simulink model "LLC2"  (R2018a)
settings: Solver=VariableStepAuto  StartTime=0.0  StopTime=0.01  RelTol=1e-3
undefined symbols (not defined in the file): Lm
libraries: powerlib x39, powerlib_meascontrol x2
settings Model: Creator=sy167  LastModifiedBy=sy167

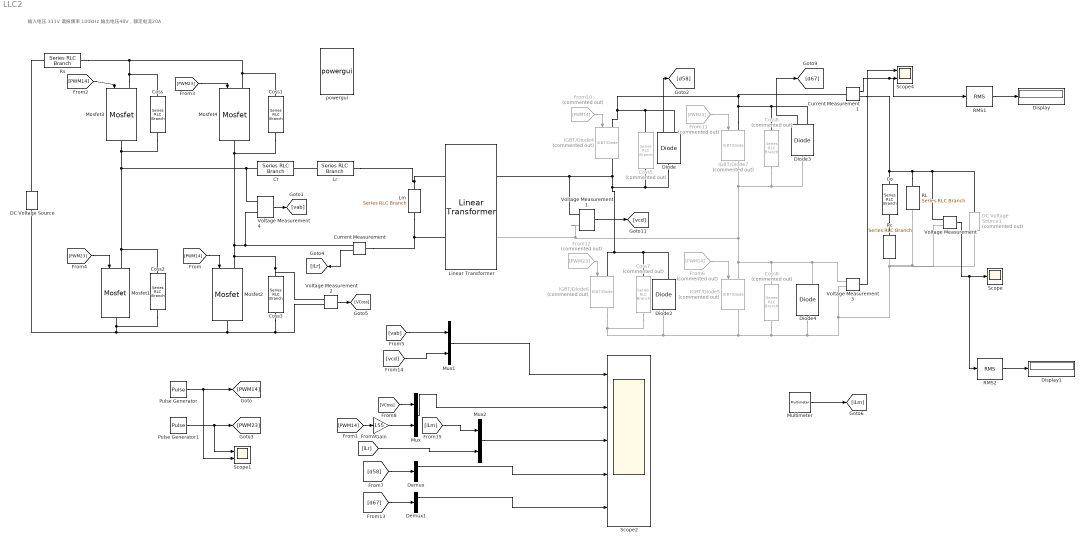
== system LLC2 ==
  note: 输入电压 311V 谐振频率 100kHz 输出电压48V，额定电流20A
  Co : powerlib/Elements/Series RLC Branch  LConnTagsString=__new0  RConnTagsString=__new0  BranchType=C  Resistance=1  Inductance=72e-6  SetiL0=off  InitialCurrent=0  Capacitance=2200e-6  Setx0=off  InitialVoltage=1500  Measurements=Branch voltage
  Coss : powerlib/Elements/Series RLC Branch  LConnTagsString=__new0  RConnTagsString=__new0  BranchType=C  Resistance=1  Inductance=72e-6  SetiL0=off  InitialCurrent=0  Capacitance=1000e-12  Setx0=off  InitialVoltage=0  Measurements=None
  Coss1 : powerlib/Elements/Series RLC Branch  LConnTagsString=__new0  RConnTagsString=__new0  BranchType=C  Resistance=1  Inductance=72e-6  SetiL0=off  InitialCurrent=0  Capacitance=1000e-12  Setx0=off  InitialVoltage=0  Measurements=None
  Coss2 : powerlib/Elements/Series RLC Branch  LConnTagsString=__new0  RConnTagsString=__new0  BranchType=C  Resistance=1  Inductance=72e-6  SetiL0=off  InitialCurrent=0  Capacitance=1000e-12  Setx0=off  InitialVoltage=0  Measurements=None
  Coss3 : powerlib/Elements/Series RLC Branch  LConnTagsString=__new0  RConnTagsString=__new0  BranchType=C  Resistance=1  Inductance=72e-6  SetiL0=off  InitialCurrent=0  Capacitance=1000e-12  Setx0=off  InitialVoltage=0  Measurements=Branch current
  Coss5 : powerlib/Elements/Series RLC Branch  Commented=on  LConnTagsString=__new0  RConnTagsString=__new0  BranchType=C  Resistance=1  Inductance=72e-6  SetiL0=off  InitialCurrent=0  Capacitance=1000e-12  Setx0=off  InitialVoltage=0  Measurements=None
  Coss6 : powerlib/Elements/Series RLC Branch  Commented=on  LConnTagsString=__new0  RConnTagsString=__new0  BranchType=C  Resistance=1  Inductance=72e-6  SetiL0=off  InitialCurrent=0  Capacitance=1000e-12  Setx0=off  InitialVoltage=0  Measurements=None
  Coss7 : powerlib/Elements/Series RLC Branch  Commented=on  LConnTagsString=__new0  RConnTagsString=__new0  BranchType=C  Resistance=1  Inductance=72e-6  SetiL0=off  InitialCurrent=0  Capacitance=1000e-12  Setx0=off  InitialVoltage=0  Measurements=None
  Coss8 : powerlib/Elements/Series RLC Branch  Commented=on  LConnTagsString=__new0  RConnTagsString=__new0  BranchType=C  Resistance=1  Inductance=72e-6  SetiL0=off  InitialCurrent=0  Capacitance=1000e-12  Setx0=off  InitialVoltage=0  Measurements=Branch current
  Cr : powerlib/Elements/Series RLC Branch  LConnTagsString=__new0  RConnTagsString=__new0  BranchType=C  Resistance=1  Inductance=72e-6  SetiL0=off  InitialCurrent=0  Capacitance=35e-9  Setx0=off  InitialVoltage=0  Measurements=None
  Current Measurement : powerlib/Measurements/Current Measurement  PhasorSimulation=off  OutputType=Complex  PSBequivalent=0
  Current Measurement1 : powerlib/Measurements/Current Measurement  PhasorSimulation=off  OutputType=Complex  PSBequivalent=0
  DC Voltage Source : powerlib/Electrical Sources/DC Voltage Source  Amplitude=311  Measurements=None
  DC Voltage Source1 : powerlib/Electrical Sources/DC Voltage Source  Commented=on  Amplitude=311  Measurements=None
  Demux : Demux  Outputs=2
  Demux1 : Demux  Outputs=2
  Diode{,2..4} (4 alike) : powerlib/Power Electronics/Diode  Ron=0.001  Lon=0  Vf=0.8  IC=0  UseSnubber=0  Rs=500  Cs=250e-9  Measurements=on
  Display : Display
  Display1 : Display
  From10 : From  Commented=on  GotoTag=PWM14
  From11 : From  Commented=on  GotoTag=PWM23
  From12 : From  Commented=on  GotoTag=PWM23
  From6 : From  Commented=on  GotoTag=PWM14
  Gain : Gain  Gain=155
  IGBT/Diode{4..7} (4 alike) : powerlib/Power Electronics/IGBT//Diode  Commented=on  Ron=1e-3  Rs=1e5  Cs=inf  Measurements=on
  Linear Transformer : powerlib/Elements/Linear Transformer  UNITS=SI  NominalPower=[ 250e6 100e3]  winding1=[6.5 0 0]  winding2=[1 0 0]  ThreeWindings=off  winding3=[1 0 0]  RmLm=[1e6 inf]  Measurements=None  DataType=on
  Lm : powerlib/Elements/Series RLC Branch  LConnTagsString=__new0  RConnTagsString=__new0  BranchType=L  Resistance=1  Inductance=146e-6  SetiL0=off  InitialCurrent=0  Capacitance=1e-6  Setx0=off  InitialVoltage=0  Measurements=Branch current
  Lr : powerlib/Elements/Series RLC Branch  LConnTagsString=__new0  RConnTagsString=__new0  BranchType=L  Resistance=1  Inductance=73e-6  SetiL0=off  InitialCurrent=0  Capacitance=1e-6  Setx0=off  InitialVoltage=0  Measurements=None
  Mosfet{1..4} (4 alike) : powerlib/Power Electronics/Mosfet  Ron=1e-3  Lon=0  Rd=0.01  Vfd=0  IC=0  Rs=1e5  Cs=inf  Measurements=off
  Multimeter : powerlib/Measurements/Multimeter  PhasorSimulation=off  OutputType=Complex  sel=3  L=4  Gain=1  yselected={'Ib: Lm'};  PSBOutputType=1  PSBequivalent=0  AxesSetting=[0,0.1,-100,100]  Display=0  SavedBlockNames=-11
  Mux : Mux  Inputs=2
  Mux1 : Mux  Inputs=2
  Mux2 : Mux  Inputs=2
  Pulse Generator : DiscretePulseGenerator  PulseType=Time based  Period=1/95e3  PulseWidth=45
  Pulse Generator1 : DiscretePulseGenerator  PulseType=Time based  Period=1/95e3  PulseWidth=45  PhaseDelay=1/95e3/2
  RL : powerlib/Elements/Series RLC Branch  LConnTagsString=__new0  RConnTagsString=__new0  BranchType=R  Resistance=48/20  Inductance=Lm  SetiL0=off  InitialCurrent=0  Capacitance=1e-6  Setx0=off  InitialVoltage=0  Measurements=None
  RMS1 : powerlib_meascontrol/Measurements/RMS  TrueRMS=on  Freq=100e3  RMSInit=120  Ts=0
  RMS2 : powerlib_meascontrol/Measurements/RMS  TrueRMS=on  Freq=100e3  RMSInit=120  Ts=0
  Rc : powerlib/Elements/Series RLC Branch  LConnTagsString=__new0  RConnTagsString=__new0  BranchType=R  Resistance=5e-3  Inductance=Lm  SetiL0=off  InitialCurrent=0  Capacitance=1e-6  Setx0=off  InitialVoltage=0  Measurements=None
  Rs : powerlib/Elements/Series RLC Branch  LConnTagsString=__new0  RConnTagsString=__new0  BranchType=R  Resistance=1e-6  Inductance=6.45e-6  SetiL0=off  InitialCurrent=0  Capacitance=1e-6  Setx0=off  InitialVoltage=0  Measurements=Branch current
  Scope : Scope
  Scope1 : Scope  NumInputPorts=2
  Scope2 : Scope  NumInputPorts=5
  Scope4 : Scope  NumInputPorts=2
  Voltage Measurement{,1..4} (5 alike) : powerlib/Measurements/Voltage Measurement  PhasorSimulation=off  OutputType=Complex  PSBequivalent=0
  powergui : powerlib/powergui  Priority=1  SimulationMode=Discrete  SampleTime=1/200e3/1000  frequency=60  Iterations=50  frequencyindice=0  Pbase=100e6  ErrMax=1e-4  UnitsV=kV  UnitsW=MW  buscounter=0  FunctionMessages=off  echomessages=off  EnableUseOfTLC=off  CurrentSourceSwitches=off  DisableSnubberDevices=off  DisableRonSwitches=off  DisableVfSwitches=off  DisplayEquations=off  SolverType=Tustin/Backward Euler (TBE)  Interpol=off  ExternalGateDelay=off  methode=off  Ts=100  x0status=blocks  SPID=off  SwTol=0  HookPort=off  RestoreLinks=warning  ResistiveCurrentMeasurement=off  Frange=[0:2:500]  Ylog=off  Xlog=on  ShowGrid=off  save=off  variable=ZData  structure=0  ZoomFFT=on  StartTime=0.0  cycles=1  DisplayStyle=1  fundamental=60  FreqAxis=off  MaxFrequency=1000  frequencyindicesteady=1  RmsSteady=1  display=off
  wires:
  Voltage Measurement/1 -> RMS2/1, Scope/1
  RMS2/1 -> Display1/1
  RMS1/1 -> Display/1
  Diode3/1 -> [d67]
  Diode/1 -> [d58]
  Voltage Measurement1/1 -> [vcd]
  Voltage Measurement3/1 -> Scope4/1
  From11/1 -> IGBT/Diode7/1
  From12/1 -> IGBT/Diode6/1
  From6/1 -> IGBT/Diode5/1
  From10/1 -> IGBT/Diode4/1
  Current Measurement1/1 -> RMS1/1, Scope4/2
  [PWM14] -> Gain/1
  [PWM14] -> Mosfet3/1
  Current Measurement/1 -> [iLr]
  Gain/1 -> Mux/2
  [PWM23] -> Mosfet1/1
  Voltage Measurement2/1 -> [VCoss]
  [PWM23] -> Mosfet4/1
  Pulse Generator/1 -> Scope1/2, [PWM14]
  Mux/1 -> Scope2/2
  Voltage Measurement4/1 -> [vab]
  Pulse Generator1/1 -> [PWM23], Scope1/1
  [VCoss] -> Mux/1
  [PWM14] -> Mosfet2/1
  [vab] -> Mux1/1
  [vcd] -> Mux1/2
  Mux1/1 -> Scope2/1
  [d58] -> Demux/1
  Demux/1 -> Scope2/4
  [d67] -> Demux1/1
  Demux1/1 -> Scope2/5
  [iLr] -> Mux2/2
  [iLm] -> Mux2/1
  Mux2/1 -> Scope2/3
  Multimeter/1 -> [iLm]
  connections:
  IGBT/Diode7/RConn1 -- Diode3/LConn1 -- Coss6/RConn1 -- Voltage Measurement1/LConn2 -- Linear Transformer/RConn2 -- Coss8/LConn1 -- Diode4/RConn1 -- Voltage Measurement3/LConn1 -- IGBT/Diode5/LConn1
  IGBT/Diode4/RConn1 -- Diode2/RConn1 -- Coss7/LConn1 -- IGBT/Diode6/LConn1 -- Diode/LConn1 -- Coss5/RConn1 -- Voltage Measurement1/LConn1 -- Linear Transformer/RConn1
  RL/LConn1 -- DC Voltage Source1/RConn1 -- Voltage Measurement/LConn1 -- Co/LConn1 -- Current Measurement1/RConn1
  Coss7/RConn1 -- IGBT/Diode5/RConn1 -- Coss8/RConn1 -- Rc/RConn1 -- RL/RConn1 -- Voltage Measurement/LConn2 -- DC Voltage Source1/LConn1 -- Voltage Measurement3/LConn2 -- Diode4/LConn1 -- Diode2/LConn1 -- IGBT/Diode6/RConn1
  IGBT/Diode7/LConn1 -- Diode3/RConn1 -- Coss6/LConn1 -- IGBT/Diode4/LConn1 -- Diode/RConn1 -- Coss5/LConn1 -- Current Measurement1/LConn1
  Co/RConn1 -- Rc/LConn1
  Current Measurement/LConn1 -- Linear Transformer/LConn2 -- Lm/RConn1
  Current Measurement/RConn1 -- Mosfet4/RConn1 -- Coss1/RConn1 -- Mosfet2/LConn1 -- Voltage Measurement2/LConn1 -- Coss3/LConn1 -- Voltage Measurement4/LConn2
  Voltage Measurement4/LConn1 -- Mosfet1/LConn1 -- Coss2/LConn1 -- Coss/RConn1 -- Mosfet3/RConn1 -- Cr/LConn1
  DC Voltage Source/LConn1 -- Mosfet2/RConn1 -- Voltage Measurement2/LConn2 -- Coss3/RConn1 -- Mosfet1/RConn1 -- Coss2/RConn1
  Lr/RConn1 -- Linear Transformer/LConn1 -- Lm/LConn1
  Mosfet3/LConn1 -- Rs/RConn1 -- Mosfet4/LConn1 -- Coss1/LConn1 -- Coss/LConn1
  DC Voltage Source/RConn1 -- Rs/LConn1
  Lr/LConn1 -- Cr/RConn1
